simulink model "Q7"  (R2021b)
settings: Solver=VariableStepAuto  StartTime=0.0  StopTime=100.0  RelTol=1e-3
undefined symbols (not defined in the file): inv_G_CL_0, K_d_LQR, K_q_LQR, K_statefeedback
settings Model: Creator=sadeg  LastModifiedBy=sadeg

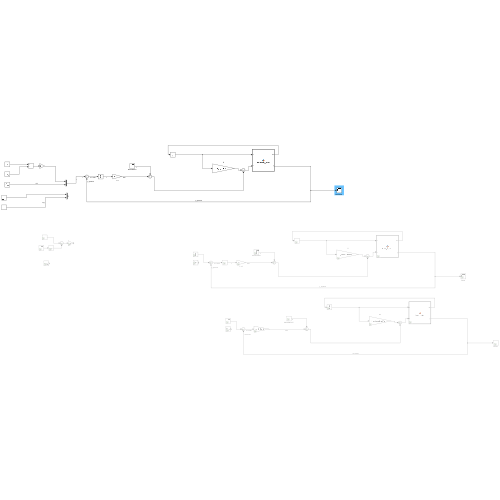
[thumbnail: Simulink's stored preview of the top-level diagram]
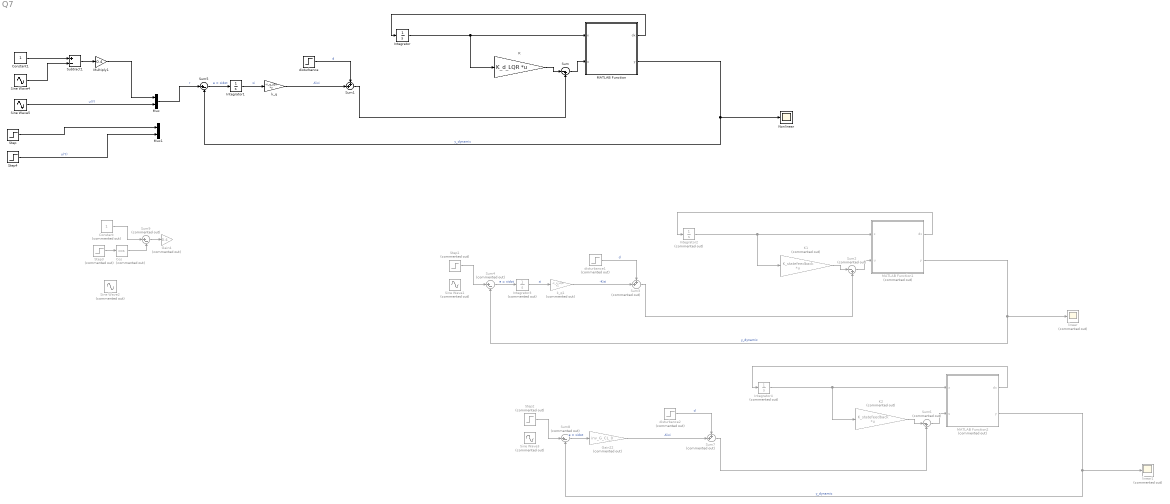
== system Q7 ==
  Constant : Constant  Commented=on
  Constant1 : Constant
  Cos : Trigonometry  Commented=on  Operator=cos
  Gain22 : Gain  Commented=on  Gain=inv_G_CL_0
  Gain4 : Gain  Commented=on  Gain=0.4
  Integrator : Integrator  InitialCondition=zeros(8,1)
  Integrator1 : Integrator
  Integrator2 : Integrator  Commented=on  InitialCondition=zeros(8,1)
  Integrator3 : Integrator  Commented=on
  Integrator4 : Integrator  Commented=on  InitialCondition=zeros(8,1)
  K : Gain  Gain=K_d_LQR  Multiplication=Matrix(K*u)
  K1 : Gain  Commented=on  Gain=K_statefeedback  Multiplication=Matrix(K*u)
  K2 : Gain  Commented=on  Gain=K_statefeedback  Multiplication=Matrix(K*u)
  MATLAB Function : MATLAB Function  TreatAsAtomicUnit=on
  MATLAB Function1 : MATLAB Function  Commented=on  TreatAsAtomicUnit=on
  MATLAB Function2 : MATLAB Function  Commented=on  TreatAsAtomicUnit=on
  Multiply1 : Gain  Gain=0.4
  Mux : Mux  Inputs=2
  Mux1 : Mux  Inputs=2
  Nonlinear : Scope
  Sine Wave1 : Sin  Commented=on  Amplitude=2  Frequency=4  SampleTime=0
  Sine Wave2 : Sin  Commented=on  Amplitude=0.4  SampleTime=0
  Sine Wave3 : Sin  Commented=on  Amplitude=2  Frequency=4  SampleTime=0
  Sine Wave4 : Sin  Phase=pi/2  SampleTime=0
  Sine Wave5 : Sin  Amplitude=0.4  SampleTime=0
  Step : Step  SampleTime=0
  Step1 : Step  Commented=on  SampleTime=0
  Step2 : Step  Commented=on  SampleTime=0
  Step3 : Step  Commented=on  Time=0  SampleTime=0
  Step4 : Step  SampleTime=0
  Subtract1 : Sum  Inputs=+-
  Sum : Sum  Inputs=|-+
  Sum1 : Sum  Inputs=++|
  Sum2 : Sum  Commented=on  Inputs=|-+
  Sum3 : Sum  Commented=on  Inputs=++|
  Sum4 : Sum  Commented=on  Inputs=|+-
  Sum5 : Sum  Inputs=|+-
  Sum6 : Sum  Commented=on  Inputs=|-+
  Sum7 : Sum  Commented=on  Inputs=++|
  Sum8 : Sum  Commented=on  Inputs=|+-
  Sum9 : Sum  Commented=on  Inputs=|+-
  disturbance : Step  Time=20  After=0.1  SampleTime=0
  disturbance1 : Step  Commented=on  Time=8  After=0.3  SampleTime=0
  disturbance2 : Step  Commented=on  Time=8  After=0.3  SampleTime=0
  k_q : Gain  Gain=-K_q_LQR  Multiplication=Matrix(K*u)
  k_q1 : Gain  Commented=on  Gain=-K_q_LQR  Multiplication=Matrix(K*u)
  linear : Scope  Commented=on
  linear1 : Scope  Commented=on
  wires:
  MATLAB Function/2(y) -> Nonlinear/1, Sum5/2  "y_dynamic"
  k_q/1 -> Sum1/2  "-Kixi"
  Integrator1/1 -> k_q/1  "xi"
  Integrator/1 -> K/1, MATLAB Function/1(x)
  Sum1/1 -> Sum/2
  Sum/1 -> MATLAB Function/2(u)
  Sum5/1 -> Integrator1/1  "e = xidot"
  MATLAB Function/1(dx) -> Integrator/1
  K/1 -> Sum/1
  disturbance/1 -> Sum1/1  "d"
  disturbance1/1 -> Sum3/1  "d"
  Integrator3/1 -> k_q1/1  "xi"
  MATLAB Function1/2(y) -> linear/1, Sum4/2  "y_dynamic"
  Sum3/1 -> Sum2/2
  k_q1/1 -> Sum3/2  "-Kixi"
  MATLAB Function1/1(dx) -> Integrator2/1
  Sum4/1 -> Integrator3/1  "e = xidot"
  Sum2/1 -> MATLAB Function1/2(u)
  Integrator2/1 -> K1/1, MATLAB Function1/1(x)
  K1/1 -> Sum2/1
  Step1/1 -> Sum4/1
  Sum6/1 -> MATLAB Function2/2(u)
  Integrator4/1 -> K2/1, MATLAB Function2/1(x)
  Step2/1 -> Sum8/1
  MATLAB Function2/1(dx) -> Integrator4/1
  Sum7/1 -> Sum6/2
  Gain22/1 -> Sum7/2  "-Kixi"
  MATLAB Function2/2(y) -> linear1/1, Sum8/2  "y_dynamic"
  disturbance2/1 -> Sum7/1  "d"
  K2/1 -> Sum6/1
  Sum8/1 -> Gain22/1  "e = xidot"
  Step3/1 -> Cos/1
  Cos/1 -> Sum9/2
  Constant/1 -> Sum9/1
  Sum9/1 -> Gain4/1
  Mux/1 -> Sum5/1  "r"
  Constant1/1 -> Subtract1/1
  Subtract1/1 -> Multiply1/1
  Sine Wave4/1 -> Subtract1/2
  Sine Wave5/1 -> Mux/2  "u(Y)"
  Multiply1/1 -> Mux/1
  Step4/1 -> Mux1/2  "u(Y)"
  Step/1 -> Mux1/1

== matlab function Q7/MATLAB Function1 ==
  data: x input size=8; u input size=2; dx output size=8; y output size=2
function [dx, y] = linear_system(x, u)

    x = reshape(x, [], 1);
    assert(length(x) == 8, 'Input x must be a vector of size 8.');


    mb = 0.11;  % mass of ball (kg)
    Jb = 1.76e-5;  % rotational moment of inertia of the ball (kgm^2)
    Rb = 0.02;  % radius of the ball (m)
    g = 9.8;  % acceleration due to gravity (m/s^2)

    % B_parameter
    B_parameter = mb / (mb + (Jb / Rb^2));

    B = [0, 0; 
         0, 0; 
         0, 0; 
         1, 0; 
         0, 0; 
         0, 0; 
         0, 0; 
         0, 1];  % 8x2 matrix

    % Nonlinear dynamics equations
    dx1 = x(2);
    dx2 = -7*x(3);
    dx3 = x(4);
    dx4 = 0;

    dx5 = x(6);
    dx6 = B_parameter * (x(5) * x(8)^2 + x(1) * x(4) * x(8) - g * sin(x(7))); %+ B(8, :) * u;  % Input influence on dx6
    dx7 = -7*x(7);
    dx8 = 0;

    % State derivative
    dx = [dx1; dx2; dx3; dx4; dx5; dx6; dx7; dx8]+ B*u;

    % Output equation: y = C*x
    C = [1, 0, 0, 0, 0, 0, 0, 0; 
         0, 0, 0, 0, 1, 0, 0, 0];  % C matrix (2x8)

    y = C * x;  % Compute the outputs
end

== matlab function Q7/MATLAB Function ==
  data: x input size=8; u input size=2; dx output size=8; y output size=2
function [dx, y] = nonlinear_system(x, u)

    x = reshape(x, [], 1);
    assert(length(x) == 8, 'Input x must be a vector of size 8.');


    mb = 0.11;  % mass of ball (kg)
    Jb = 1.76e-5;  % rotational moment of inertia of the ball (kgm^2)
    Rb = 0.02;  % radius of the ball (m)
    g = 9.8;  % acceleration due to gravity (m/s^2)

    % B_parameter
    B_parameter = mb / (mb + (Jb / Rb^2));

    B = [0, 0; 
         0, 0; 
         0, 0; 
         1, 0; 
         0, 0; 
         0, 0; 
         0, 0; 
         0, 1];  % 8x2 matrix

    % Nonlinear dynamics equations
    dx1 = x(2);
    dx2 = B_parameter * (x(1) * x(4)^2 + x(4) * x(5) * x(8) - g * sin(x(3))); %+ B(4, :) * u;  % Input influence on dx2
    dx3 = x(4);
    dx4 = 0;

    dx5 = x(6);
    dx6 = B_parameter * (x(5) * x(8)^2 + x(1) * x(4) * x(8) - g * sin(x(7))); %+ B(8, :) * u;  % Input influence on dx6
    dx7 = x(8);
    dx8 = 0;

    % State derivative
    dx = [dx1; dx2; dx3; dx4; dx5; dx6; dx7; dx8]+ B*u;

    % Output equation: y = C*x
    C = [1, 0, 0, 0, 0, 0, 0, 0; 
         0, 0, 0, 0, 1, 0, 0, 0];  % C matrix (2x8)

    y = C * x;  % Compute the outputs
end

== matlab function Q7/MATLAB Function2 ==
  data: x input size=8; u input size=2; dx output size=8; y output size=2
function [dx, y] = linear_system(x, u)

    x = reshape(x, [], 1);
    assert(length(x) == 8, 'Input x must be a vector of size 8.');


    mb = 0.11;  % mass of ball (kg)
    Jb = 1.76e-5;  % rotational moment of inertia of the ball (kgm^2)
    Rb = 0.02;  % radius of the ball (m)
    g = 9.8;  % acceleration due to gravity (m/s^2)

    % B_parameter
    B_parameter = mb / (mb + (Jb / Rb^2));

    B = [0, 0; 
         0, 0; 
         0, 0; 
         1, 0; 
         0, 0; 
         0, 0; 
         0, 0; 
         0, 1];  % 8x2 matrix

    % Nonlinear dynamics equations
    dx1 = x(2);
    dx2 = -7*x(3);
    dx3 = x(4);
    dx4 = 0;

    dx5 = x(6);
    dx6 = B_parameter * (x(5) * x(8)^2 + x(1) * x(4) * x(8) - g * sin(x(7))); %+ B(8, :) * u;  % Input influence on dx6
    dx7 = -7*x(7);
    dx8 = 0;

    % State derivative
    dx = [dx1; dx2; dx3; dx4; dx5; dx6; dx7; dx8]+ B*u;

    % Output equation: y = C*x
    C = [1, 0, 0, 0, 0, 0, 0, 0; 
         0, 0, 0, 0, 1, 0, 0, 0];  % C matrix (2x8)

    y = C * x;  % Compute the outputs
end
